simulink model "2_PID_tuning"  (R2015b)
settings: Solver=VariableStepAuto  StartTime=0.0  StopTime=10  RelTol=1e-3
values from neighbouring files (symbols this model uses):
  g = 9.8    [1_CB_simulation_paremeter.m]    (also in matlab_cycle_bot.m = 9.81; simulation_paremeter.m)
  Ib = (1/12)* mb * (Lb^2)    (= 0.0002316)    [1_CB_simulation_paremeter.m]    (also in simulation_paremeter.m)
  It = ((Iw)+(mw*Lw))+((Ib)+(mb*Lb))    (= 0.0644941)    [1_CB_simulation_paremeter.m]    (also in simulation_paremeter.m)
  Iw = ((1/2)*mw*(r^2))+ (Mring * r *r)    (= 0.0003425)    [1_CB_simulation_paremeter.m]    (also in simulation_paremeter.m)
  Kb = 0.0116    [1_CB_simulation_paremeter.m]    (also in matlab_cycle_bot.m = 0.0115833333333; simulation_paremeter.m)
  Kt = 0.0116    [1_CB_simulation_paremeter.m]    (also in matlab_cycle_bot.m = 0.0115833333333; simulation_paremeter.m)
  Lb = 0.06    [1_CB_simulation_paremeter.m]    (also in simulation_paremeter.m)
  Lw = 0.1    [1_CB_simulation_paremeter.m]    (also in simulation_paremeter.m)
  mb = 0.772    [1_CB_simulation_paremeter.m]    (also in simulation_paremeter.m)
  mw = 0.176    [1_CB_simulation_paremeter.m]    (also in matlab_cycle_bot.m; simulation_paremeter.m)
  R = 4.5    [1_CB_simulation_paremeter.m]    (also in matlab_cycle_bot.m = 0.15; simulation_paremeter.m)
libraries: simulink x3, dspsrcs4 x1
settings Model: Creator=prit varmora  LastModifiedBy=prit varmora

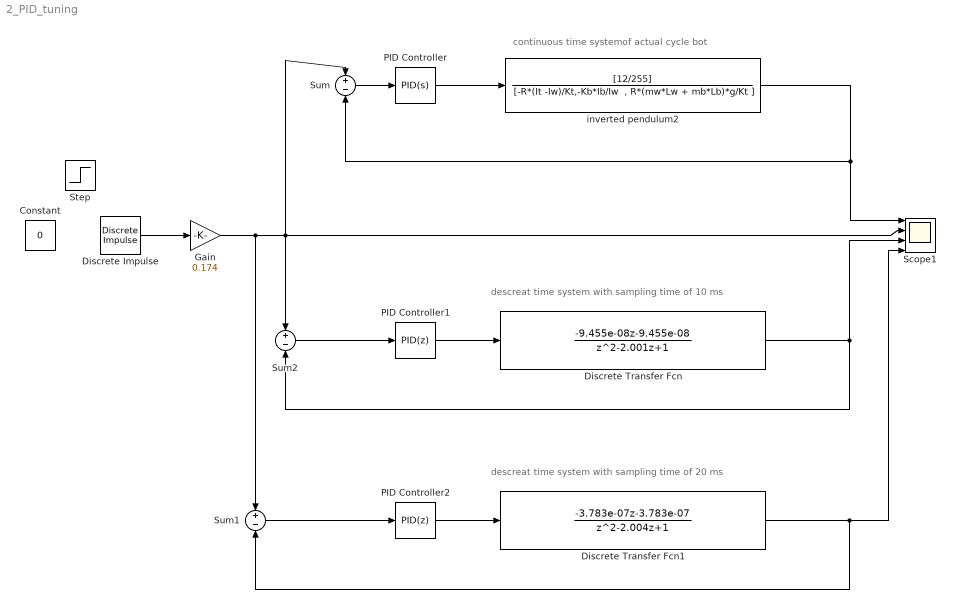
== system 2_PID_tuning ==
  note: descreat time system with sampling time of 10 ms
  note: continuous time systemof actual cycle bot
  note: descreat time system with sampling time of 20 ms
  Constant : Constant  Value=0
  Discrete Transfer Fcn : DiscreteTransferFcn  Numerator=|  Denominator=[1 ,-2.001 , +1]  SampleTime=0.01
      | [  
      |   -9.455e-08 , 
      |   -9.455e-08]
  Discrete Transfer Fcn1 : DiscreteTransferFcn  Numerator="[  -3.783e-07, -3.783e-07]"  Denominator=[1 ,-2.004 , +1]
  Discrete Impulse : dspsrcs4/Discrete  Impulse  Delay=2  SampleTime=0.2  FrameSample=1  OutputFrames=off  dataType=double  isSigned=on  wordLen=16  udDataType=sfix(16)  fracBitsMode=Best precision  numFracBits=15  OutDataTypeStr=double  LastOutDataTypeStr=double
  Gain : Gain  Gain=0.174
  PID Controller : simulink/Continuous/PID Controller  Controller=PID  TimeDomain=Continuous-time  SampleTime=-1  IntegratorMethod=Forward Euler  FilterMethod=Forward Euler  Form=Parallel  UseFilter=on  ControllerParametersSource=internal  P=-14793.8088998622  I=-7153.08182665227  D=-7649.03810240291  N=3167.09334937223  InitialConditionSource=internal  InitialConditionForIntegrator=0  InitialConditionForFilter=0  ExternalReset=none  LimitOutput=off  UpperSaturationLimit=inf  LowerSaturationLimit=-inf  LinearizeAsGain=on  AntiWindupMode=none  Kb=1  TrackingMode=off  Kt=1  PParamMin=[]  PParamMax=[]  IParamMin=[]  IParamMax=[]  DParamMin=[]  DParamMax=[]  NParamMin=[]  NParamMax=[]  KbParamMin=[]  KbParamMax=[]  KtParamMin=[]  KtParamMax=[]  POutMin=[]  POutMax=[]  IOutMin=[]  IOutMax=[]  DOutMin=[]  DOutMax=[]  NOutMin=[]  NOutMax=[]  KbOutMin=[]  KbOutMax=[]  KtOutMin=[]  KtOutMax=[]  IntegratorOutMin=[]  IntegratorOutMax=[]  FilterOutMin=[]  FilterOutMax=[]  SumOutMin=[]  SumOutMax=[]  SumI1OutMin=[]  SumI1OutMax=[]  SumI2OutMin=[]  SumI2OutMax=[]  SumI3OutMin=[]  SumI3OutMax=[]  SumDOutMin=[]  SumDOutMax=[]  SaturationOutMin=[]  SaturationOutMax=[]  IntegratorContinuousStateAttributes=''  IntegratorStateMustResolveToSignalObject=off  IntegratorRTWStateStorageClass=Auto  FilterContinuousStateAttributes=''  FilterStateMustResolveToSignalObject=off  FilterRTWStateStorageClass=Auto  DifferentiatorICPrevScaledInput=0  DifferentiatorOutMin=[]  DifferentiatorOutMax=[]
  PID Controller1 : simulink/Continuous/PID Controller  Controller=PID  TimeDomain=Discrete-time  SampleTime=0.01  IntegratorMethod=Forward Euler  FilterMethod=Forward Euler  Form=Parallel  UseFilter=off  ControllerParametersSource=internal  P=-14793.8088998622  I=-7153.08182665227  D=-7649.03810240291  N=3167.09334937223  InitialConditionSource=internal  InitialConditionForIntegrator=0  InitialConditionForFilter=0  ExternalReset=none  LimitOutput=off  UpperSaturationLimit=inf  LowerSaturationLimit=-inf  LinearizeAsGain=on  AntiWindupMode=none  Kb=1  TrackingMode=off  Kt=1  PParamMin=[]  PParamMax=[]  IParamMin=[]  IParamMax=[]  DParamMin=[]  DParamMax=[]  NParamMin=[]  NParamMax=[]  KbParamMin=[]  KbParamMax=[]  KtParamMin=[]  KtParamMax=[]  POutMin=[]  POutMax=[]  IOutMin=[]  IOutMax=[]  DOutMin=[]  DOutMax=[]  NOutMin=[]  NOutMax=[]  KbOutMin=[]  KbOutMax=[]  KtOutMin=[]  KtOutMax=[]  IntegratorOutMin=[]  IntegratorOutMax=[]  FilterOutMin=[]  FilterOutMax=[]  SumOutMin=[]  SumOutMax=[]  SumI1OutMin=[]  SumI1OutMax=[]  SumI2OutMin=[]  SumI2OutMax=[]  SumI3OutMin=[]  SumI3OutMax=[]  SumDOutMin=[]  SumDOutMax=[]  SaturationOutMin=[]  SaturationOutMax=[]  IntegratorContinuousStateAttributes=''  IntegratorStateMustResolveToSignalObject=off  IntegratorRTWStateStorageClass=Auto  FilterContinuousStateAttributes=''  FilterStateMustResolveToSignalObject=off  FilterRTWStateStorageClass=Auto  DifferentiatorICPrevScaledInput=0  DifferentiatorOutMin=[]  DifferentiatorOutMax=[]
  PID Controller2 : simulink/Continuous/PID Controller  Controller=PID  TimeDomain=Discrete-time  SampleTime=0.02  IntegratorMethod=Forward Euler  FilterMethod=Forward Euler  Form=Parallel  UseFilter=off  ControllerParametersSource=internal  P=-14793.8088998622  I=-7153.08182665227  D=-7649.03810240291  N=3167.09334937223  InitialConditionSource=internal  InitialConditionForIntegrator=0  InitialConditionForFilter=0  ExternalReset=none  LimitOutput=off  UpperSaturationLimit=inf  LowerSaturationLimit=-inf  LinearizeAsGain=on  AntiWindupMode=none  Kb=1  TrackingMode=off  Kt=1  PParamMin=[]  PParamMax=[]  IParamMin=[]  IParamMax=[]  DParamMin=[]  DParamMax=[]  NParamMin=[]  NParamMax=[]  KbParamMin=[]  KbParamMax=[]  KtParamMin=[]  KtParamMax=[]  POutMin=[]  POutMax=[]  IOutMin=[]  IOutMax=[]  DOutMin=[]  DOutMax=[]  NOutMin=[]  NOutMax=[]  KbOutMin=[]  KbOutMax=[]  KtOutMin=[]  KtOutMax=[]  IntegratorOutMin=[]  IntegratorOutMax=[]  FilterOutMin=[]  FilterOutMax=[]  SumOutMin=[]  SumOutMax=[]  SumI1OutMin=[]  SumI1OutMax=[]  SumI2OutMin=[]  SumI2OutMax=[]  SumI3OutMin=[]  SumI3OutMax=[]  SumDOutMin=[]  SumDOutMax=[]  SaturationOutMin=[]  SaturationOutMax=[]  IntegratorContinuousStateAttributes=''  IntegratorStateMustResolveToSignalObject=off  IntegratorRTWStateStorageClass=Auto  FilterContinuousStateAttributes=''  FilterStateMustResolveToSignalObject=off  FilterRTWStateStorageClass=Auto  DifferentiatorICPrevScaledInput=0  DifferentiatorOutMin=[]  DifferentiatorOutMax=[]
  Scope1 : Scope  NumInputPorts=4
  Step : Step  SampleTime=0
  Sum : Sum  Inputs=+-
  Sum1 : Sum  Inputs=+-
  Sum2 : Sum  Inputs=+-
  inverted pendulum2 : TransferFcn  Numerator=[12/255]  Denominator="[-R*(It -Iw)/Kt,-Kb*Ib/Iw  , R*(mw*Lw + mb*Lb)*g/Kt ]"  ContinuousStateAttributes='pendulam_inclination'
  wires:
  Sum/1 -> PID Controller/1
  inverted pendulum2/1 -> Scope1/1, Sum/2
  PID Controller1/1 -> Discrete Transfer Fcn/1
  Sum2/1 -> PID Controller1/1
  Discrete Impulse/1 -> Gain/1
  PID Controller/1 -> inverted pendulum2/1
  PID Controller2/1 -> Discrete Transfer Fcn1/1
  Discrete Transfer Fcn1/1 -> Scope1/4, Sum1/2
  Sum1/1 -> PID Controller2/1
  Discrete Transfer Fcn/1 -> Scope1/3, Sum2/2
  Gain/1 -> Sum/1, Scope1/2, Sum2/1, Sum1/1
